simulink model "lab_1"  (R2023a)
settings: Solver=VariableStepAuto  StartTime=0.0  StopTime=60  RelTol=1e-3
settings Model: Creator=User  LastModifiedBy=User

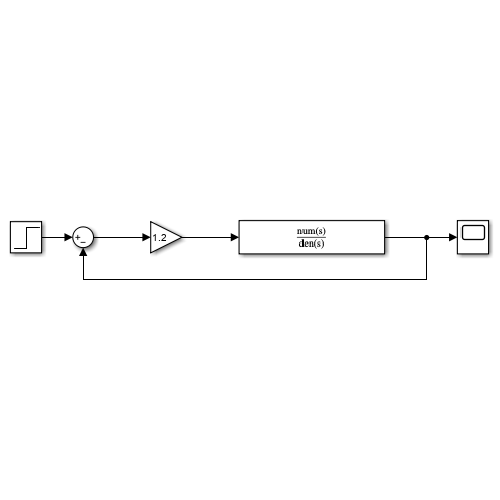
[thumbnail: Simulink's stored preview of the top-level diagram]
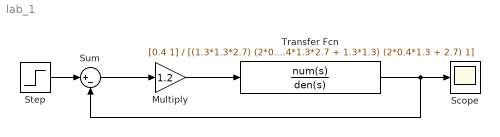
== system lab_1 ==
  Multiply : Gain  Gain=1.2
  Scope : Scope
  Step : Step  SampleTime=0
  Sum : Sum  Inputs=|+-
  Transfer Fcn : TransferFcn  Numerator=[0.4 1]  Denominator=[(1.3*1.3*2.7) (2*0.4*1.3*2.7 + 1.3*1.3) (2*0.4*1.3 + 2.7) 1]
  wires:
  Step/1 -> Sum/1
  Transfer Fcn/1 -> Sum/2, Scope/1
  Sum/1 -> Multiply/1
  Multiply/1 -> Transfer Fcn/1
